simulink model "TSR_Scenario_005_cs"  (R2014b)
settings: Solver=ode5  SolverMode=SingleTasking  StartTime=0.0  StopTime=inf  FixedStep=1/100  RelTol=1e-3
PreLoadFcn:
  | mbxruntime.callbacks.PreLoadFcn(bdroot);
  | check_NUTS_defined;
  | 
  | assignin('base',['model_closed_' bdroot],false);
  | 
  | addpath('../includes_TSR/includes_TSR');
  | 
  | switch version('-release')
  | case {'2010a', '2010b', '2011a'}
  | addpath('../includes_TSR/ML2010b');
  | otherwise
  | addpath('../includes_TSR/ML2011b');
  | end
PostLoadFcn:
  | mbxruntime.callbacks.PostLoadFcn(bdroot);
InitFcn:
  | mbxruntime.callbacks.InitFcn(bdroot);
StartFcn:
  | mbxruntime.callbacks.StartFcn(bdroot);
StopFcn:
  | mbxruntime.callbacks.StopFcn(bdroot);
model workspace: external: MAT-File .\TSR_Scenario_005_cs_hws.mat (data not in the file)
undefined symbols (not defined in the file or in its folder): InitImageOutputDir, mbxruntime, OrientationPitch, OrientationRoll, PositionX, PositionY, PositionZ, tabledata, warningInitialVelocity, x0
undefined symbols (not defined in the file): SteeringColumn, SteeringWheel, TSR_Scenario_005_cs_00431f954bf6ed0a, TSR_Scenario_005_cs_02a6645fe307ce96, TSR_Scenario_005_cs_0e0d17e780cba748, TSR_Scenario_005_cs_0f94700004e304be, TSR_Scenario_005_cs_13e63084604f23c5, TSR_Scenario_005_cs_18da76569b226b1d, TSR_Scenario_005_cs_19a09eb0dceaf389, TSR_Scenario_005_cs_1d6b1ecf339da803, TSR_Scenario_005_cs_219485daa5a5d171, TSR_Scenario_005_cs_221c03cfb0670d1a, TSR_Scenario_005_cs_22611db63f83df91, TSR_Scenario_005_cs_24324341e1f0fdeb, TSR_Scenario_005_cs_248b5be6aaeb4a32, TSR_Scenario_005_cs_26d69342f02903e6, TSR_Scenario_005_cs_28d4639b4eb6a924, TSR_Scenario_005_cs_2a50646ef6121283, TSR_Scenario_005_cs_2addef8764f78195, TSR_Scenario_005_cs_2c78bb6e92f1c73d, TSR_Scenario_005_cs_330b013c7926b8c0, TSR_Scenario_005_cs_33ac55a3a4bfafc5, TSR_Scenario_005_cs_33d6442482a921b6, TSR_Scenario_005_cs_36fcc85960c1dc31, TSR_Scenario_005_cs_38acb22310967a91, TSR_Scenario_005_cs_3e8855054a9c05f5, TSR_Scenario_005_cs_43d01b44652f0f38, TSR_Scenario_005_cs_43d19ecb630bd754, TSR_Scenario_005_cs_4487c76a87b8c5f1, TSR_Scenario_005_cs_44ceee846c318dfb, TSR_Scenario_005_cs_450a3683cbfdd730, TSR_Scenario_005_cs_464618e49e37493a, TSR_Scenario_005_cs_4880b38df4698ab1, TSR_Scenario_005_cs_4a2b3c7d0abca22e, TSR_Scenario_005_cs_4bd204b8239d5406, TSR_Scenario_005_cs_4de8d67ffbf74a19, TSR_Scenario_005_cs_4f6170ee339e194e, TSR_Scenario_005_cs_50430c8166448bfc, TSR_Scenario_005_cs_53c8f6734eaacbd2, TSR_Scenario_005_cs_543db9a2ff458ebe, TSR_Scenario_005_cs_57976f30ab2edad5, TSR_Scenario_005_cs_5922fccf31372278, TSR_Scenario_005_cs_5a258c940bbe826b, TSR_Scenario_005_cs_6087cc283675db35, TSR_Scenario_005_cs_6246b869963d4acb, TSR_Scenario_005_cs_6352b9f9b72630f9, TSR_Scenario_005_cs_6559b64eceddc3ca, TSR_Scenario_005_cs_6832a8ea8fa66aa4, TSR_Scenario_005_cs_696d53dba69844e5, TSR_Scenario_005_cs_6cabbb37c4ac2dd1, TSR_Scenario_005_cs_6d528aa494c8a952, TSR_Scenario_005_cs_6d945b49f7234fd2, TSR_Scenario_005_cs_6e2ebc771acb2455, TSR_Scenario_005_cs_7897f864ad990cf0, TSR_Scenario_005_cs_7978c65fd141f076, TSR_Scenario_005_cs_7a9ba94120bbe2c7, TSR_Scenario_005_cs_7b108592703c2dc5, TSR_Scenario_005_cs_7cd2f5b09394b811, TSR_Scenario_005_cs_7e1904d085d8f37f, TSR_Scenario_005_cs_7e555208507e0618 ... (+95)
libraries: simulink_extras x59, PreScanSimulinkLibrary x43, simulink x29
(part 19 of 24)

== system TSR_Scenario_005_cs/Audi_A8_1/WheelDisplacement_Mux/WheelR0_Mux ==
  X [m] : Inport
  Y [m] : Inport  Port=2
  Z [m] : Inport  Port=3
  Roll [rad] : Inport  Port=4
  Pitch [rad] : Inport  Port=5
  Yaw [rad] : Inport  Port=6
  Bus Creator : BusCreator  Inputs=3  OutDataTypeStr=Bus: PRESCAN_XYZ_DATA
  Bus Creator1 : BusCreator  Inputs=3  OutDataTypeStr=Bus: PRESCAN_RPY_DATA
  Bus Creator2 : BusCreator  Inputs=2  OutDataTypeStr=Bus: PRESCAN_POSE_DATA
  Joint : Outport
  wires:
  Yaw [rad]/1 -> Bus Creator1/3  "Yaw"
  Bus Creator1/1 -> Bus Creator2/2  "ORIENTATION"
  Bus Creator/1 -> Bus Creator2/1  "POSITION"
  X [m]/1 -> Bus Creator/1  "X"
  Y [m]/1 -> Bus Creator/2  "Y"
  Z [m]/1 -> Bus Creator/3  "Z"
  Bus Creator2/1 -> Joint/1
  Roll [rad]/1 -> Bus Creator1/1  "Roll"
  Pitch [rad]/1 -> Bus Creator1/2  "Pitch"

== system TSR_Scenario_005_cs/Audi_A8_1/WheelDisplacement_Mux/WheelR1_Mux ==
  X [m] : Inport
  Y [m] : Inport  Port=2
  Z [m] : Inport  Port=3
  Roll [rad] : Inport  Port=4
  Pitch [rad] : Inport  Port=5
  Yaw [rad] : Inport  Port=6
  Bus Creator : BusCreator  Inputs=3  OutDataTypeStr=Bus: PRESCAN_XYZ_DATA
  Bus Creator1 : BusCreator  Inputs=3  OutDataTypeStr=Bus: PRESCAN_RPY_DATA
  Bus Creator2 : BusCreator  Inputs=2  OutDataTypeStr=Bus: PRESCAN_POSE_DATA
  Joint : Outport
  wires:
  Yaw [rad]/1 -> Bus Creator1/3  "Yaw"
  Bus Creator1/1 -> Bus Creator2/2  "ORIENTATION"
  Bus Creator/1 -> Bus Creator2/1  "POSITION"
  X [m]/1 -> Bus Creator/1  "X"
  Y [m]/1 -> Bus Creator/2  "Y"
  Z [m]/1 -> Bus Creator/3  "Z"
  Bus Creator2/1 -> Joint/1
  Roll [rad]/1 -> Bus Creator1/1  "Roll"
  Pitch [rad]/1 -> Bus Creator1/2  "Pitch"

== system TSR_Scenario_005_cs/BMW_X5_1/Dynamics_Empty/MuxState ==
  note: mode: Dynamics
  note: mode: Positioning
  note: mode: Dynamics
      | VelVEHICLE
      | wrt VEH
  note: AnglesVEHICLE
      | wrtGLOB
  note: For state mode 'Dynamic' positions
      | are not taken into account, as they
      | are computed by integrating velocity.
      | Click annotation for Help.
  x [m] : Inport  SampleTime=TimeStep
  y [m] : Inport  Port=2  SampleTime=TimeStep
  z [m] : Inport  Port=3  SampleTime=TimeStep
  dx [m/s] : Inport  Port=4  SampleTime=TimeStep
  dy [m/s] : Inport  Port=5  SampleTime=TimeStep
  dz [m/s] : Inport  Port=6  SampleTime=TimeStep
  R [rad] : Inport  Port=7  SampleTime=TimeStep
  P [rad] : Inport  Port=8  SampleTime=TimeStep
  Y [rad] : Inport  Port=9  SampleTime=TimeStep
  Constant : Constant  DisableCoverage=on  Value=positioningmode
  Discrete-Time Integrator : DiscreteIntegrator  SampleTime=TimeStep
  Ground : Ground
  Ground1 : Ground
  Mux1 : Mux  Inputs=[3 3]
  Mux2 : Mux  Inputs=3
  Mux3 : Mux  Inputs=3
  Mux4 : Mux  Inputs=3
  Mux5 : Mux  Inputs=[3 3]
  Mux6 : Mux  Inputs=[6 3]
  Switch : Switch  Threshold=0.5
  Transformation_BODY2GLOBAL : PreScanSimulinkLibrary/Simple_Vehicle_Dynamics/Chassis/MuxDynState/Transformation_BODY2GLOBAL
  mux3 : Mux  Inputs=3
  state : Outport
  wires:
  Constant/1 -> Switch/2
  Mux6/1 -> state/1
  Mux4/1 -> Mux1/1
  Mux5/1 -> Switch/3
  Mux1/1 -> Switch/1
  Switch/1 -> Mux6/1  "PosVeh wrt  GLOB"
  P [rad]/1 -> Mux3/2
  R [rad]/1 -> Mux3/1
  dz [m/s]/1 -> Mux2/3
  dy [m/s]/1 -> Mux2/2
  dx [m/s]/1 -> Mux2/1
  z [m]/1 -> Mux4/3
  y [m]/1 -> Mux4/2
  x [m]/1 -> Mux4/1
  Ground1/1 -> mux3/2  "pitch"
  Y [rad]/1 -> mux3/3, Mux3/3  "yaw"
  Mux3/1 -> Mux6/2
  Transformation_BODY2GLOBAL/1 -> Discrete-Time Integrator/1, Mux5/2  "VelVEH wrt  GLOB"
  mux3/1 -> Transformation_BODY2GLOBAL/2
  Ground/1 -> mux3/1  "roll"
  Mux2/1 -> Mux1/2, Transformation_BODY2GLOBAL/1
  Discrete-Time Integrator/1 -> Mux5/1  "PosVEH wrt  GLOB"

== system TSR_Scenario_005_cs/BMW_X5_1/Dynamics_Empty/STATE_BMW_X5_1 ==
  State : Inport  SampleTime=TimeStep
  Bus Creator : BusCreator  Inputs=15  OutDataTypeStr=Bus: PRESCAN_STATEACTUATORDATA  NonVirtualBus=on
  Constant : Constant  Value=0
  Demux : Demux  Outputs=15
  Mux : Mux  Inputs=3
  Mux1 : Mux  Inputs=3
  Mux2 : Mux  Inputs=3
  iniBODYAngles wrtVEH [rad] : Constant  Value=Roll0  SampleTime=TimeStep
  iniBODYAngles wrtVEH [rad]1 : Constant  Value=Pitch0  SampleTime=TimeStep
  iniVEHAngles wrtGLOB [rad] : Constant  Value=Yaw0  SampleTime=TimeStep
  iniVEHposition wrtGLOB [m] : Constant  Value=x0  SampleTime=TimeStep
  iniVEHposition wrtGLOB [m]1 : Constant  Value=y0  SampleTime=TimeStep
  iniVEHposition wrtGLOB [m]2 : Constant  Value=z0  SampleTime=TimeStep
  state2FullState : PreScanSimulinkLibrary/state2FullState  SystemSampleTime=-1
  StateBus : Outport  OutDataTypeStr=Bus: PRESCAN_STATEACTUATORDATA
  wires:
  Mux2/1 -> state2FullState/4
  iniVEHAngles wrtGLOB [rad]/1 -> Mux2/3
  Mux1/1 -> state2FullState/3
  Constant/1 -> Mux2/1, Mux2/2, Mux1/3
  iniBODYAngles wrtVEH [rad]1/1 -> Mux1/2
  iniBODYAngles wrtVEH [rad]/1 -> Mux1/1
  Mux/1 -> state2FullState/2
  iniVEHposition wrtGLOB [m]2/1 -> Mux/3
  iniVEHposition wrtGLOB [m]/1 -> Mux/1
  iniVEHposition wrtGLOB [m]1/1 -> Mux/2
  Demux/15 -> Bus Creator/15  "AngularVelocityYaw"
  Demux/14 -> Bus Creator/14  "AngularVelocityPitch"
  Demux/13 -> Bus Creator/13  "AngularVelocityRoll"
  Demux/12 -> Bus Creator/12  "OrientationYaw"
  Demux/11 -> Bus Creator/11  "OrientationPitch"
  Demux/10 -> Bus Creator/10  "OrientationRoll"
  Demux/9 -> Bus Creator/9  "AccelerationZ"
  Demux/8 -> Bus Creator/8  "AccelerationY"
  Demux/7 -> Bus Creator/7  "AccelerationX"
  Demux/6 -> Bus Creator/6  "VelocityZ"
  Demux/5 -> Bus Creator/5  "VelocityY"
  Demux/4 -> Bus Creator/4  "VelocityX"
  Demux/3 -> Bus Creator/3  "PositionZ"
  Demux/2 -> Bus Creator/2  "PositionY"
  Demux/1 -> Bus Creator/1  "PositionX"
  state2FullState/1 -> Demux/1
  State/1 -> state2FullState/1
  Bus Creator/1 -> StateBus/1

== system TSR_Scenario_005_cs/BMW_X5_1/SELF_Demux/compas converter ==
  rotz [rad] : Inport
  cart2compas : Subsystem
  rad2deg : Gain  Gain=180/pi
  heading [deg] : Outport
  wires:
  rad2deg/1 -> cart2compas/1(Angle [deg])
  rotz [rad]/1 -> rad2deg/1
  cart2compas/1(heading [deg]) -> heading [deg]/1

== system TSR_Scenario_005_cs/BMW_X5_2/Dynamics_Empty/MuxState ==
  note: mode: Dynamics
  note: mode: Positioning
  note: mode: Dynamics
      | VelVEHICLE
      | wrt VEH
  note: AnglesVEHICLE
      | wrtGLOB
  note: For state mode 'Dynamic' positions
      | are not taken into account, as they
      | are computed by integrating velocity.
      | Click annotation for Help.
  x [m] : Inport  SampleTime=TimeStep
  y [m] : Inport  Port=2  SampleTime=TimeStep
  z [m] : Inport  Port=3  SampleTime=TimeStep
  dx [m/s] : Inport  Port=4  SampleTime=TimeStep
  dy [m/s] : Inport  Port=5  SampleTime=TimeStep
  dz [m/s] : Inport  Port=6  SampleTime=TimeStep
  R [rad] : Inport  Port=7  SampleTime=TimeStep
  P [rad] : Inport  Port=8  SampleTime=TimeStep
  Y [rad] : Inport  Port=9  SampleTime=TimeStep
  Constant : Constant  DisableCoverage=on  Value=positioningmode
  Discrete-Time Integrator : DiscreteIntegrator  SampleTime=TimeStep
  Ground : Ground
  Ground1 : Ground
  Mux1 : Mux  Inputs=[3 3]
  Mux2 : Mux  Inputs=3
  Mux3 : Mux  Inputs=3
  Mux4 : Mux  Inputs=3
  Mux5 : Mux  Inputs=[3 3]
  Mux6 : Mux  Inputs=[6 3]
  Switch : Switch  Threshold=0.5
  Transformation_BODY2GLOBAL : PreScanSimulinkLibrary/Simple_Vehicle_Dynamics/Chassis/MuxDynState/Transformation_BODY2GLOBAL
  mux3 : Mux  Inputs=3
  state : Outport
  wires:
  Constant/1 -> Switch/2
  Mux6/1 -> state/1
  Mux4/1 -> Mux1/1
  Mux5/1 -> Switch/3
  Mux1/1 -> Switch/1
  Switch/1 -> Mux6/1  "PosVeh wrt  GLOB"
  P [rad]/1 -> Mux3/2
  R [rad]/1 -> Mux3/1
  dz [m/s]/1 -> Mux2/3
  dy [m/s]/1 -> Mux2/2
  dx [m/s]/1 -> Mux2/1
  z [m]/1 -> Mux4/3
  y [m]/1 -> Mux4/2
  x [m]/1 -> Mux4/1
  Ground1/1 -> mux3/2  "pitch"
  Y [rad]/1 -> mux3/3, Mux3/3  "yaw"
  Mux3/1 -> Mux6/2
  Transformation_BODY2GLOBAL/1 -> Discrete-Time Integrator/1, Mux5/2  "VelVEH wrt  GLOB"
  mux3/1 -> Transformation_BODY2GLOBAL/2
  Ground/1 -> mux3/1  "roll"
  Mux2/1 -> Mux1/2, Transformation_BODY2GLOBAL/1
  Discrete-Time Integrator/1 -> Mux5/1  "PosVEH wrt  GLOB"

== system TSR_Scenario_005_cs/BMW_X5_2/Dynamics_Empty/STATE_BMW_X5_2 ==
  State : Inport  SampleTime=TimeStep
  Bus Creator : BusCreator  Inputs=15  OutDataTypeStr=Bus: PRESCAN_STATEACTUATORDATA  NonVirtualBus=on
  Constant : Constant  Value=0
  Demux : Demux  Outputs=15
  Mux : Mux  Inputs=3
  Mux1 : Mux  Inputs=3
  Mux2 : Mux  Inputs=3
  iniBODYAngles wrtVEH [rad] : Constant  Value=Roll0  SampleTime=TimeStep
  iniBODYAngles wrtVEH [rad]1 : Constant  Value=Pitch0  SampleTime=TimeStep
  iniVEHAngles wrtGLOB [rad] : Constant  Value=Yaw0  SampleTime=TimeStep
  iniVEHposition wrtGLOB [m] : Constant  Value=x0  SampleTime=TimeStep
  iniVEHposition wrtGLOB [m]1 : Constant  Value=y0  SampleTime=TimeStep
  iniVEHposition wrtGLOB [m]2 : Constant  Value=z0  SampleTime=TimeStep
  state2FullState : PreScanSimulinkLibrary/state2FullState  SystemSampleTime=-1
  StateBus : Outport  OutDataTypeStr=Bus: PRESCAN_STATEACTUATORDATA
  wires:
  Mux2/1 -> state2FullState/4
  iniVEHAngles wrtGLOB [rad]/1 -> Mux2/3
  Mux1/1 -> state2FullState/3
  Constant/1 -> Mux2/1, Mux2/2, Mux1/3
  iniBODYAngles wrtVEH [rad]1/1 -> Mux1/2
  iniBODYAngles wrtVEH [rad]/1 -> Mux1/1
  Mux/1 -> state2FullState/2
  iniVEHposition wrtGLOB [m]2/1 -> Mux/3
  iniVEHposition wrtGLOB [m]/1 -> Mux/1
  iniVEHposition wrtGLOB [m]1/1 -> Mux/2
  Demux/15 -> Bus Creator/15  "AngularVelocityYaw"
  Demux/14 -> Bus Creator/14  "AngularVelocityPitch"
  Demux/13 -> Bus Creator/13  "AngularVelocityRoll"
  Demux/12 -> Bus Creator/12  "OrientationYaw"
  Demux/11 -> Bus Creator/11  "OrientationPitch"
  Demux/10 -> Bus Creator/10  "OrientationRoll"
  Demux/9 -> Bus Creator/9  "AccelerationZ"
  Demux/8 -> Bus Creator/8  "AccelerationY"
  Demux/7 -> Bus Creator/7  "AccelerationX"
  Demux/6 -> Bus Creator/6  "VelocityZ"
  Demux/5 -> Bus Creator/5  "VelocityY"
  Demux/4 -> Bus Creator/4  "VelocityX"
  Demux/3 -> Bus Creator/3  "PositionZ"
  Demux/2 -> Bus Creator/2  "PositionY"
  Demux/1 -> Bus Creator/1  "PositionX"
  state2FullState/1 -> Demux/1
  State/1 -> state2FullState/1
  Bus Creator/1 -> StateBus/1

== system TSR_Scenario_005_cs/BMW_X5_2/SELF_Demux/compas converter ==
  rotz [rad] : Inport
  cart2compas : Subsystem
  rad2deg : Gain  Gain=180/pi
  heading [deg] : Outport
  wires:
  rad2deg/1 -> cart2compas/1(Angle [deg])
  rotz [rad]/1 -> rad2deg/1
  cart2compas/1(heading [deg]) -> heading [deg]/1

== system TSR_Scenario_005_cs/BMW_X5_3/Dynamics_Empty/MuxState ==
  note: mode: Dynamics
  note: mode: Positioning
  note: mode: Dynamics
      | VelVEHICLE
      | wrt VEH
  note: AnglesVEHICLE
      | wrtGLOB
  note: For state mode 'Dynamic' positions
      | are not taken into account, as they
      | are computed by integrating velocity.
      | Click annotation for Help.
  x [m] : Inport  SampleTime=TimeStep
  y [m] : Inport  Port=2  SampleTime=TimeStep
  z [m] : Inport  Port=3  SampleTime=TimeStep
  dx [m/s] : Inport  Port=4  SampleTime=TimeStep
  dy [m/s] : Inport  Port=5  SampleTime=TimeStep
  dz [m/s] : Inport  Port=6  SampleTime=TimeStep
  R [rad] : Inport  Port=7  SampleTime=TimeStep
  P [rad] : Inport  Port=8  SampleTime=TimeStep
  Y [rad] : Inport  Port=9  SampleTime=TimeStep
  Constant : Constant  DisableCoverage=on  Value=positioningmode
  Discrete-Time Integrator : DiscreteIntegrator  SampleTime=TimeStep
  Ground : Ground
  Ground1 : Ground
  Mux1 : Mux  Inputs=[3 3]
  Mux2 : Mux  Inputs=3
  Mux3 : Mux  Inputs=3
  Mux4 : Mux  Inputs=3
  Mux5 : Mux  Inputs=[3 3]
  Mux6 : Mux  Inputs=[6 3]
  Switch : Switch  Threshold=0.5
  Transformation_BODY2GLOBAL : PreScanSimulinkLibrary/Simple_Vehicle_Dynamics/Chassis/MuxDynState/Transformation_BODY2GLOBAL
  mux3 : Mux  Inputs=3
  state : Outport
  wires:
  Constant/1 -> Switch/2
  Mux6/1 -> state/1
  Mux4/1 -> Mux1/1
  Mux5/1 -> Switch/3
  Mux1/1 -> Switch/1
  Switch/1 -> Mux6/1  "PosVeh wrt  GLOB"
  P [rad]/1 -> Mux3/2
  R [rad]/1 -> Mux3/1
  dz [m/s]/1 -> Mux2/3
  dy [m/s]/1 -> Mux2/2
  dx [m/s]/1 -> Mux2/1
  z [m]/1 -> Mux4/3
  y [m]/1 -> Mux4/2
  x [m]/1 -> Mux4/1
  Ground1/1 -> mux3/2  "pitch"
  Y [rad]/1 -> mux3/3, Mux3/3  "yaw"
  Mux3/1 -> Mux6/2
  Transformation_BODY2GLOBAL/1 -> Discrete-Time Integrator/1, Mux5/2  "VelVEH wrt  GLOB"
  mux3/1 -> Transformation_BODY2GLOBAL/2
  Ground/1 -> mux3/1  "roll"
  Mux2/1 -> Mux1/2, Transformation_BODY2GLOBAL/1
  Discrete-Time Integrator/1 -> Mux5/1  "PosVEH wrt  GLOB"

== system TSR_Scenario_005_cs/BMW_X5_3/Dynamics_Empty/STATE_BMW_X5_3 ==
  State : Inport  SampleTime=TimeStep
  Bus Creator : BusCreator  Inputs=15  OutDataTypeStr=Bus: PRESCAN_STATEACTUATORDATA  NonVirtualBus=on
  Constant : Constant  Value=0
  Demux : Demux  Outputs=15
  Mux : Mux  Inputs=3
  Mux1 : Mux  Inputs=3
  Mux2 : Mux  Inputs=3
  iniBODYAngles wrtVEH [rad] : Constant  Value=Roll0  SampleTime=TimeStep
  iniBODYAngles wrtVEH [rad]1 : Constant  Value=Pitch0  SampleTime=TimeStep
  iniVEHAngles wrtGLOB [rad] : Constant  Value=Yaw0  SampleTime=TimeStep
  iniVEHposition wrtGLOB [m] : Constant  Value=x0  SampleTime=TimeStep
  iniVEHposition wrtGLOB [m]1 : Constant  Value=y0  SampleTime=TimeStep
  iniVEHposition wrtGLOB [m]2 : Constant  Value=z0  SampleTime=TimeStep
  state2FullState : PreScanSimulinkLibrary/state2FullState  SystemSampleTime=-1
  StateBus : Outport  OutDataTypeStr=Bus: PRESCAN_STATEACTUATORDATA
  wires:
  Mux2/1 -> state2FullState/4
  iniVEHAngles wrtGLOB [rad]/1 -> Mux2/3
  Mux1/1 -> state2FullState/3
  Constant/1 -> Mux2/1, Mux2/2, Mux1/3
  iniBODYAngles wrtVEH [rad]1/1 -> Mux1/2
  iniBODYAngles wrtVEH [rad]/1 -> Mux1/1
  Mux/1 -> state2FullState/2
  iniVEHposition wrtGLOB [m]2/1 -> Mux/3
  iniVEHposition wrtGLOB [m]/1 -> Mux/1
  iniVEHposition wrtGLOB [m]1/1 -> Mux/2
  Demux/15 -> Bus Creator/15  "AngularVelocityYaw"
  Demux/14 -> Bus Creator/14  "AngularVelocityPitch"
  Demux/13 -> Bus Creator/13  "AngularVelocityRoll"
  Demux/12 -> Bus Creator/12  "OrientationYaw"
  Demux/11 -> Bus Creator/11  "OrientationPitch"
  Demux/10 -> Bus Creator/10  "OrientationRoll"
  Demux/9 -> Bus Creator/9  "AccelerationZ"
  Demux/8 -> Bus Creator/8  "AccelerationY"
  Demux/7 -> Bus Creator/7  "AccelerationX"
  Demux/6 -> Bus Creator/6  "VelocityZ"
  Demux/5 -> Bus Creator/5  "VelocityY"
  Demux/4 -> Bus Creator/4  "VelocityX"
  Demux/3 -> Bus Creator/3  "PositionZ"
  Demux/2 -> Bus Creator/2  "PositionY"
  Demux/1 -> Bus Creator/1  "PositionX"
  state2FullState/1 -> Demux/1
  State/1 -> state2FullState/1
  Bus Creator/1 -> StateBus/1

== system TSR_Scenario_005_cs/BMW_X5_3/SELF_Demux/compas converter ==
  rotz [rad] : Inport
  cart2compas : Subsystem
  rad2deg : Gain  Gain=180/pi
  heading [deg] : Outport
  wires:
  rad2deg/1 -> cart2compas/1(Angle [deg])
  rotz [rad]/1 -> rad2deg/1
  cart2compas/1(heading [deg]) -> heading [deg]/1

== system TSR_Scenario_005_cs/BMW_Z3_1/Dynamics_Empty/MuxState ==
  note: mode: Dynamics
  note: mode: Positioning
  note: mode: Dynamics
      | VelVEHICLE
      | wrt VEH
  note: AnglesVEHICLE
      | wrtGLOB
  note: For state mode 'Dynamic' positions
      | are not taken into account, as they
      | are computed by integrating velocity.
      | Click annotation for Help.
  x [m] : Inport  SampleTime=TimeStep
  y [m] : Inport  Port=2  SampleTime=TimeStep
  z [m] : Inport  Port=3  SampleTime=TimeStep
  dx [m/s] : Inport  Port=4  SampleTime=TimeStep
  dy [m/s] : Inport  Port=5  SampleTime=TimeStep
  dz [m/s] : Inport  Port=6  SampleTime=TimeStep
  R [rad] : Inport  Port=7  SampleTime=TimeStep
  P [rad] : Inport  Port=8  SampleTime=TimeStep
  Y [rad] : Inport  Port=9  SampleTime=TimeStep
  Constant : Constant  DisableCoverage=on  Value=positioningmode
  Discrete-Time Integrator : DiscreteIntegrator  SampleTime=TimeStep
  Ground : Ground
  Ground1 : Ground
  Mux1 : Mux  Inputs=[3 3]
  Mux2 : Mux  Inputs=3
  Mux3 : Mux  Inputs=3
  Mux4 : Mux  Inputs=3
  Mux5 : Mux  Inputs=[3 3]
  Mux6 : Mux  Inputs=[6 3]
  Switch : Switch  Threshold=0.5
  Transformation_BODY2GLOBAL : PreScanSimulinkLibrary/Simple_Vehicle_Dynamics/Chassis/MuxDynState/Transformation_BODY2GLOBAL
  mux3 : Mux  Inputs=3
  state : Outport
  wires:
  Constant/1 -> Switch/2
  Mux6/1 -> state/1
  Mux4/1 -> Mux1/1
  Mux5/1 -> Switch/3
  Mux1/1 -> Switch/1
  Switch/1 -> Mux6/1  "PosVeh wrt  GLOB"
  P [rad]/1 -> Mux3/2
  R [rad]/1 -> Mux3/1
  dz [m/s]/1 -> Mux2/3
  dy [m/s]/1 -> Mux2/2
  dx [m/s]/1 -> Mux2/1
  z [m]/1 -> Mux4/3
  y [m]/1 -> Mux4/2
  x [m]/1 -> Mux4/1
  Ground1/1 -> mux3/2  "pitch"
  Y [rad]/1 -> mux3/3, Mux3/3  "yaw"
  Mux3/1 -> Mux6/2
  Transformation_BODY2GLOBAL/1 -> Discrete-Time Integrator/1, Mux5/2  "VelVEH wrt  GLOB"
  mux3/1 -> Transformation_BODY2GLOBAL/2
  Ground/1 -> mux3/1  "roll"
  Mux2/1 -> Mux1/2, Transformation_BODY2GLOBAL/1
  Discrete-Time Integrator/1 -> Mux5/1  "PosVEH wrt  GLOB"

== system TSR_Scenario_005_cs/BMW_Z3_1/Dynamics_Empty/STATE_BMW_Z3_1 ==
  State : Inport  SampleTime=TimeStep
  Bus Creator : BusCreator  Inputs=15  OutDataTypeStr=Bus: PRESCAN_STATEACTUATORDATA  NonVirtualBus=on
  Constant : Constant  Value=0
  Demux : Demux  Outputs=15
  Mux : Mux  Inputs=3
  Mux1 : Mux  Inputs=3
  Mux2 : Mux  Inputs=3
  iniBODYAngles wrtVEH [rad] : Constant  Value=Roll0  SampleTime=TimeStep
  iniBODYAngles wrtVEH [rad]1 : Constant  Value=Pitch0  SampleTime=TimeStep
  iniVEHAngles wrtGLOB [rad] : Constant  Value=Yaw0  SampleTime=TimeStep
  iniVEHposition wrtGLOB [m] : Constant  Value=x0  SampleTime=TimeStep
  iniVEHposition wrtGLOB [m]1 : Constant  Value=y0  SampleTime=TimeStep
  iniVEHposition wrtGLOB [m]2 : Constant  Value=z0  SampleTime=TimeStep
  state2FullState : PreScanSimulinkLibrary/state2FullState  SystemSampleTime=-1
  StateBus : Outport  OutDataTypeStr=Bus: PRESCAN_STATEACTUATORDATA
  wires:
  Mux2/1 -> state2FullState/4
  iniVEHAngles wrtGLOB [rad]/1 -> Mux2/3
  Mux1/1 -> state2FullState/3
  Constant/1 -> Mux2/1, Mux2/2, Mux1/3
  iniBODYAngles wrtVEH [rad]1/1 -> Mux1/2
  iniBODYAngles wrtVEH [rad]/1 -> Mux1/1
  Mux/1 -> state2FullState/2
  iniVEHposition wrtGLOB [m]2/1 -> Mux/3
  iniVEHposition wrtGLOB [m]/1 -> Mux/1
  iniVEHposition wrtGLOB [m]1/1 -> Mux/2
  Demux/15 -> Bus Creator/15  "AngularVelocityYaw"
  Demux/14 -> Bus Creator/14  "AngularVelocityPitch"
  Demux/13 -> Bus Creator/13  "AngularVelocityRoll"
  Demux/12 -> Bus Creator/12  "OrientationYaw"
  Demux/11 -> Bus Creator/11  "OrientationPitch"
  Demux/10 -> Bus Creator/10  "OrientationRoll"
  Demux/9 -> Bus Creator/9  "AccelerationZ"
  Demux/8 -> Bus Creator/8  "AccelerationY"
  Demux/7 -> Bus Creator/7  "AccelerationX"
  Demux/6 -> Bus Creator/6  "VelocityZ"
  Demux/5 -> Bus Creator/5  "VelocityY"
  Demux/4 -> Bus Creator/4  "VelocityX"
  Demux/3 -> Bus Creator/3  "PositionZ"
  Demux/2 -> Bus Creator/2  "PositionY"
  Demux/1 -> Bus Creator/1  "PositionX"
  state2FullState/1 -> Demux/1
  State/1 -> state2FullState/1
  Bus Creator/1 -> StateBus/1

== system TSR_Scenario_005_cs/BMW_Z3_1/SELF_Demux/compas converter ==
  rotz [rad] : Inport
  cart2compas : Subsystem
  rad2deg : Gain  Gain=180/pi
  heading [deg] : Outport
  wires:
  rad2deg/1 -> cart2compas/1(Angle [deg])
  rotz [rad]/1 -> rad2deg/1
  cart2compas/1(heading [deg]) -> heading [deg]/1

== system TSR_Scenario_005_cs/CarTrailer_SingleAxle_1/SELF_Demux/compas converter ==
  rotz [rad] : Inport
  cart2compas : Subsystem
  rad2deg : Gain  Gain=180/pi
  heading [deg] : Outport
  wires:
  rad2deg/1 -> cart2compas/1(Angle [deg])
  rotz [rad]/1 -> rad2deg/1
  cart2compas/1(heading [deg]) -> heading [deg]/1

== system TSR_Scenario_005_cs/Citroen_C3_1/Dynamics_Empty/MuxState ==
  note: mode: Dynamics
  note: mode: Positioning
  note: mode: Dynamics
      | VelVEHICLE
      | wrt VEH
  note: AnglesVEHICLE
      | wrtGLOB
  note: For state mode 'Dynamic' positions
      | are not taken into account, as they
      | are computed by integrating velocity.
      | Click annotation for Help.
  x [m] : Inport  SampleTime=TimeStep
  y [m] : Inport  Port=2  SampleTime=TimeStep
  z [m] : Inport  Port=3  SampleTime=TimeStep
  dx [m/s] : Inport  Port=4  SampleTime=TimeStep
  dy [m/s] : Inport  Port=5  SampleTime=TimeStep
  dz [m/s] : Inport  Port=6  SampleTime=TimeStep
  R [rad] : Inport  Port=7  SampleTime=TimeStep
  P [rad] : Inport  Port=8  SampleTime=TimeStep
  Y [rad] : Inport  Port=9  SampleTime=TimeStep
  Constant : Constant  DisableCoverage=on  Value=positioningmode
  Discrete-Time Integrator : DiscreteIntegrator  SampleTime=TimeStep
  Ground : Ground
  Ground1 : Ground
  Mux1 : Mux  Inputs=[3 3]
  Mux2 : Mux  Inputs=3
  Mux3 : Mux  Inputs=3
  Mux4 : Mux  Inputs=3
  Mux5 : Mux  Inputs=[3 3]
  Mux6 : Mux  Inputs=[6 3]
  Switch : Switch  Threshold=0.5
  Transformation_BODY2GLOBAL : PreScanSimulinkLibrary/Simple_Vehicle_Dynamics/Chassis/MuxDynState/Transformation_BODY2GLOBAL
  mux3 : Mux  Inputs=3
  state : Outport
  wires:
  Constant/1 -> Switch/2
  Mux6/1 -> state/1
  Mux4/1 -> Mux1/1
  Mux5/1 -> Switch/3
  Mux1/1 -> Switch/1
  Switch/1 -> Mux6/1  "PosVeh wrt  GLOB"
  P [rad]/1 -> Mux3/2
  R [rad]/1 -> Mux3/1
  dz [m/s]/1 -> Mux2/3
  dy [m/s]/1 -> Mux2/2
  dx [m/s]/1 -> Mux2/1
  z [m]/1 -> Mux4/3
  y [m]/1 -> Mux4/2
  x [m]/1 -> Mux4/1
  Ground1/1 -> mux3/2  "pitch"
  Y [rad]/1 -> mux3/3, Mux3/3  "yaw"
  Mux3/1 -> Mux6/2
  Transformation_BODY2GLOBAL/1 -> Discrete-Time Integrator/1, Mux5/2  "VelVEH wrt  GLOB"
  mux3/1 -> Transformation_BODY2GLOBAL/2
  Ground/1 -> mux3/1  "roll"
  Mux2/1 -> Mux1/2, Transformation_BODY2GLOBAL/1
  Discrete-Time Integrator/1 -> Mux5/1  "PosVEH wrt  GLOB"

== system TSR_Scenario_005_cs/Citroen_C3_1/Dynamics_Empty/STATE_Citroen_C3_1 ==
  State : Inport  SampleTime=TimeStep
  Bus Creator : BusCreator  Inputs=15  OutDataTypeStr=Bus: PRESCAN_STATEACTUATORDATA  NonVirtualBus=on
  Constant : Constant  Value=0
  Demux : Demux  Outputs=15
  Mux : Mux  Inputs=3
  Mux1 : Mux  Inputs=3
  Mux2 : Mux  Inputs=3
  iniBODYAngles wrtVEH [rad] : Constant  Value=Roll0  SampleTime=TimeStep
  iniBODYAngles wrtVEH [rad]1 : Constant  Value=Pitch0  SampleTime=TimeStep
  iniVEHAngles wrtGLOB [rad] : Constant  Value=Yaw0  SampleTime=TimeStep
  iniVEHposition wrtGLOB [m] : Constant  Value=x0  SampleTime=TimeStep
  iniVEHposition wrtGLOB [m]1 : Constant  Value=y0  SampleTime=TimeStep
  iniVEHposition wrtGLOB [m]2 : Constant  Value=z0  SampleTime=TimeStep
  state2FullState : PreScanSimulinkLibrary/state2FullState  SystemSampleTime=-1
  StateBus : Outport  OutDataTypeStr=Bus: PRESCAN_STATEACTUATORDATA
  wires:
  Mux2/1 -> state2FullState/4
  iniVEHAngles wrtGLOB [rad]/1 -> Mux2/3
  Mux1/1 -> state2FullState/3
  Constant/1 -> Mux2/1, Mux2/2, Mux1/3
  iniBODYAngles wrtVEH [rad]1/1 -> Mux1/2
  iniBODYAngles wrtVEH [rad]/1 -> Mux1/1
  Mux/1 -> state2FullState/2
  iniVEHposition wrtGLOB [m]2/1 -> Mux/3
  iniVEHposition wrtGLOB [m]/1 -> Mux/1
  iniVEHposition wrtGLOB [m]1/1 -> Mux/2
  Demux/15 -> Bus Creator/15  "AngularVelocityYaw"
  Demux/14 -> Bus Creator/14  "AngularVelocityPitch"
  Demux/13 -> Bus Creator/13  "AngularVelocityRoll"
  Demux/12 -> Bus Creator/12  "OrientationYaw"
  Demux/11 -> Bus Creator/11  "OrientationPitch"
  Demux/10 -> Bus Creator/10  "OrientationRoll"
  Demux/9 -> Bus Creator/9  "AccelerationZ"
  Demux/8 -> Bus Creator/8  "AccelerationY"
  Demux/7 -> Bus Creator/7  "AccelerationX"
  Demux/6 -> Bus Creator/6  "VelocityZ"
  Demux/5 -> Bus Creator/5  "VelocityY"
  Demux/4 -> Bus Creator/4  "VelocityX"
  Demux/3 -> Bus Creator/3  "PositionZ"
  Demux/2 -> Bus Creator/2  "PositionY"
  Demux/1 -> Bus Creator/1  "PositionX"
  state2FullState/1 -> Demux/1
  State/1 -> state2FullState/1
  Bus Creator/1 -> StateBus/1

== system TSR_Scenario_005_cs/Citroen_C3_1/SELF_Demux/compas converter ==
  rotz [rad] : Inport
  cart2compas : Subsystem
  rad2deg : Gain  Gain=180/pi
  heading [deg] : Outport
  wires:
  rad2deg/1 -> cart2compas/1(Angle [deg])
  rotz [rad]/1 -> rad2deg/1
  cart2compas/1(heading [deg]) -> heading [deg]/1

== system TSR_Scenario_005_cs/Daf_95_1/SELF_Demux/compas converter ==
  rotz [rad] : Inport
  cart2compas : Subsystem
  rad2deg : Gain  Gain=180/pi
  heading [deg] : Outport
  wires:
  rad2deg/1 -> cart2compas/1(Angle [deg])
  rotz [rad]/1 -> rad2deg/1
  cart2compas/1(heading [deg]) -> heading [deg]/1

== system TSR_Scenario_005_cs/Female_RegularAni_1/Animation/animation mode ==
  vel : Inport
  Data Type Conversion : DataTypeConversion  OutDataTypeStr=double
  Fcn : Fcn  Expr=sqrt(u(1)^2+u(2)^2+u(3)^2)
  Running : simulink/Logic and Bit Operations/Compare To Constant  relop=>=  const=MWS  OutDataTypeStr=uint8  ZeroCross=off
  Sum : Sum  Inputs=|++
  Walking : simulink/Logic and Bit Operations/Compare To Zero  relop=~=  OutDataTypeStr=uint8  ZeroCross=off
  mode : Outport
  wires:
  vel/1 -> Fcn/1
  Sum/1 -> Data Type Conversion/1
  Walking/1 -> Sum/1
  Running/1 -> Sum/2
  Fcn/1 -> Walking/1, Running/1
  Data Type Conversion/1 -> mode/1

== system TSR_Scenario_005_cs/Female_RegularAni_1/Animation/elapsed track ==
  vel : Inport
  Discrete-Time Integrator : DiscreteIntegrator  SampleTime=-1
  Fcn : Fcn  Expr=sqrt(u(1)^2 + u(2)^2 + u(3)^2)
  s : Outport
  wires:
  Fcn/1 -> Discrete-Time Integrator/1
  vel/1 -> Fcn/1
  Discrete-Time Integrator/1 -> s/1

== system TSR_Scenario_005_cs/Female_RegularAni_1/SELF_Demux/compas converter ==
  rotz [rad] : Inport
  cart2compas : Subsystem
  rad2deg : Gain  Gain=180/pi
  heading [deg] : Outport
  wires:
  rad2deg/1 -> cart2compas/1(Angle [deg])
  rotz [rad]/1 -> rad2deg/1
  cart2compas/1(heading [deg]) -> heading [deg]/1

== system TSR_Scenario_005_cs/Female_Regular_wBuggy_1/Animation/animation mode ==
  vel : Inport
  Data Type Conversion : DataTypeConversion  OutDataTypeStr=int32
  Fcn : Fcn  Expr=u(1)^2+u(2)^2+u(3)^2
  Walking : simulink/Logic and Bit Operations/Compare To Zero  relop=~=  OutDataTypeStr=uint8  ZeroCross=off
  mode : Outport
  wires:
  Data Type Conversion/1 -> mode/1
  Walking/1 -> Data Type Conversion/1
  Fcn/1 -> Walking/1
  vel/1 -> Fcn/1

== system TSR_Scenario_005_cs/Female_Regular_wBuggy_1/Animation/elapsed track ==
  vel : Inport
  Discrete-Time Integrator : DiscreteIntegrator  SampleTime=-1
  Fcn : Fcn  Expr=sqrt(u(1)^2 + u(2)^2 + u(3)^2)
  s : Outport
  wires:
  Discrete-Time Integrator/1 -> s/1
  vel/1 -> Fcn/1
  Fcn/1 -> Discrete-Time Integrator/1

== system TSR_Scenario_005_cs/Female_Regular_wBuggy_1/Dynamics_Empty/MuxState ==
  note: mode: Dynamics
  note: mode: Positioning
  note: mode: Dynamics
      | VelVEHICLE
      | wrt VEH
  note: AnglesVEHICLE
      | wrtGLOB
  note: For state mode 'Dynamic' positions
      | are not taken into account, as they
      | are computed by integrating velocity.
      | Click annotation for Help.
  x [m] : Inport  SampleTime=TimeStep
  y [m] : Inport  Port=2  SampleTime=TimeStep
  z [m] : Inport  Port=3  SampleTime=TimeStep
  dx [m/s] : Inport  Port=4  SampleTime=TimeStep
  dy [m/s] : Inport  Port=5  SampleTime=TimeStep
  dz [m/s] : Inport  Port=6  SampleTime=TimeStep
  R [rad] : Inport  Port=7  SampleTime=TimeStep
  P [rad] : Inport  Port=8  SampleTime=TimeStep
  Y [rad] : Inport  Port=9  SampleTime=TimeStep
  Constant : Constant  DisableCoverage=on  Value=positioningmode
  Discrete-Time Integrator : DiscreteIntegrator  SampleTime=TimeStep
  Ground : Ground
  Ground1 : Ground
  Mux1 : Mux  Inputs=[3 3]
  Mux2 : Mux  Inputs=3
  Mux3 : Mux  Inputs=3
  Mux4 : Mux  Inputs=3
  Mux5 : Mux  Inputs=[3 3]
  Mux6 : Mux  Inputs=[6 3]
  Switch : Switch  Threshold=0.5
  Transformation_BODY2GLOBAL : PreScanSimulinkLibrary/Simple_Vehicle_Dynamics/Chassis/MuxDynState/Transformation_BODY2GLOBAL
  mux3 : Mux  Inputs=3
  state : Outport
  wires:
  Constant/1 -> Switch/2
  Mux6/1 -> state/1
  Mux4/1 -> Mux1/1
  Mux5/1 -> Switch/3
  Mux1/1 -> Switch/1
  Switch/1 -> Mux6/1  "PosVeh wrt  GLOB"
  P [rad]/1 -> Mux3/2
  R [rad]/1 -> Mux3/1
  dz [m/s]/1 -> Mux2/3
  dy [m/s]/1 -> Mux2/2
  dx [m/s]/1 -> Mux2/1
  z [m]/1 -> Mux4/3
  y [m]/1 -> Mux4/2
  x [m]/1 -> Mux4/1
  Ground1/1 -> mux3/2  "pitch"
  Y [rad]/1 -> mux3/3, Mux3/3  "yaw"
  Mux3/1 -> Mux6/2
  Transformation_BODY2GLOBAL/1 -> Discrete-Time Integrator/1, Mux5/2  "VelVEH wrt  GLOB"
  mux3/1 -> Transformation_BODY2GLOBAL/2
  Ground/1 -> mux3/1  "roll"
  Mux2/1 -> Mux1/2, Transformation_BODY2GLOBAL/1
  Discrete-Time Integrator/1 -> Mux5/1  "PosVEH wrt  GLOB"

== system TSR_Scenario_005_cs/Female_Regular_wBuggy_1/Dynamics_Empty/STATE_Female_Regular_wBuggy_1 ==
  State : Inport  SampleTime=TimeStep
  Bus Creator : BusCreator  Inputs=15  OutDataTypeStr=Bus: PRESCAN_STATEACTUATORDATA  NonVirtualBus=on
  Constant : Constant  Value=0
  Demux : Demux  Outputs=15
  Mux : Mux  Inputs=3
  Mux1 : Mux  Inputs=3
  Mux2 : Mux  Inputs=3
  iniBODYAngles wrtVEH [rad] : Constant  Value=Roll0  SampleTime=TimeStep
  iniBODYAngles wrtVEH [rad]1 : Constant  Value=Pitch0  SampleTime=TimeStep
  iniVEHAngles wrtGLOB [rad] : Constant  Value=Yaw0  SampleTime=TimeStep
  iniVEHposition wrtGLOB [m] : Constant  Value=x0  SampleTime=TimeStep
  iniVEHposition wrtGLOB [m]1 : Constant  Value=y0  SampleTime=TimeStep
  iniVEHposition wrtGLOB [m]2 : Constant  Value=z0  SampleTime=TimeStep
  state2FullState : PreScanSimulinkLibrary/state2FullState  SystemSampleTime=-1
  StateBus : Outport  OutDataTypeStr=Bus: PRESCAN_STATEACTUATORDATA
  wires:
  Mux2/1 -> state2FullState/4
  iniVEHAngles wrtGLOB [rad]/1 -> Mux2/3
  Mux1/1 -> state2FullState/3
  Constant/1 -> Mux2/1, Mux2/2, Mux1/3
  iniBODYAngles wrtVEH [rad]1/1 -> Mux1/2
  iniBODYAngles wrtVEH [rad]/1 -> Mux1/1
  Mux/1 -> state2FullState/2
  iniVEHposition wrtGLOB [m]2/1 -> Mux/3
  iniVEHposition wrtGLOB [m]/1 -> Mux/1
  iniVEHposition wrtGLOB [m]1/1 -> Mux/2
  Demux/15 -> Bus Creator/15  "AngularVelocityYaw"
  Demux/14 -> Bus Creator/14  "AngularVelocityPitch"
  Demux/13 -> Bus Creator/13  "AngularVelocityRoll"
  Demux/12 -> Bus Creator/12  "OrientationYaw"
  Demux/11 -> Bus Creator/11  "OrientationPitch"
  Demux/10 -> Bus Creator/10  "OrientationRoll"
  Demux/9 -> Bus Creator/9  "AccelerationZ"
  Demux/8 -> Bus Creator/8  "AccelerationY"
  Demux/7 -> Bus Creator/7  "AccelerationX"
  Demux/6 -> Bus Creator/6  "VelocityZ"
  Demux/5 -> Bus Creator/5  "VelocityY"
  Demux/4 -> Bus Creator/4  "VelocityX"
  Demux/3 -> Bus Creator/3  "PositionZ"
  Demux/2 -> Bus Creator/2  "PositionY"
  Demux/1 -> Bus Creator/1  "PositionX"
  state2FullState/1 -> Demux/1
  State/1 -> state2FullState/1
  Bus Creator/1 -> StateBus/1

== system TSR_Scenario_005_cs/Female_Regular_wBuggy_1/SELF_Demux/compas converter ==
  rotz [rad] : Inport
  cart2compas : Subsystem
  rad2deg : Gain  Gain=180/pi
  heading [deg] : Outport
  wires:
  rad2deg/1 -> cart2compas/1(Angle [deg])
  rotz [rad]/1 -> rad2deg/1
  cart2compas/1(heading [deg]) -> heading [deg]/1

== system TSR_Scenario_005_cs/Fiat_Bravo_1/Dynamics_Empty/MuxState ==
  note: mode: Dynamics
  note: mode: Positioning
  note: mode: Dynamics
      | VelVEHICLE
      | wrt VEH
  note: AnglesVEHICLE
      | wrtGLOB
  note: For state mode 'Dynamic' positions
      | are not taken into account, as they
      | are computed by integrating velocity.
      | Click annotation for Help.
  x [m] : Inport  SampleTime=TimeStep
  y [m] : Inport  Port=2  SampleTime=TimeStep
  z [m] : Inport  Port=3  SampleTime=TimeStep
  dx [m/s] : Inport  Port=4  SampleTime=TimeStep
  dy [m/s] : Inport  Port=5  SampleTime=TimeStep
  dz [m/s] : Inport  Port=6  SampleTime=TimeStep
  R [rad] : Inport  Port=7  SampleTime=TimeStep
  P [rad] : Inport  Port=8  SampleTime=TimeStep
  Y [rad] : Inport  Port=9  SampleTime=TimeStep
  Constant : Constant  DisableCoverage=on  Value=positioningmode
  Discrete-Time Integrator : DiscreteIntegrator  SampleTime=TimeStep
  Ground : Ground
  Ground1 : Ground
  Mux1 : Mux  Inputs=[3 3]
  Mux2 : Mux  Inputs=3
  Mux3 : Mux  Inputs=3
  Mux4 : Mux  Inputs=3
  Mux5 : Mux  Inputs=[3 3]
  Mux6 : Mux  Inputs=[6 3]
  Switch : Switch  Threshold=0.5
  Transformation_BODY2GLOBAL : PreScanSimulinkLibrary/Simple_Vehicle_Dynamics/Chassis/MuxDynState/Transformation_BODY2GLOBAL
  mux3 : Mux  Inputs=3
  state : Outport
  wires:
  Constant/1 -> Switch/2
  Mux6/1 -> state/1
  Mux4/1 -> Mux1/1
  Mux5/1 -> Switch/3
  Mux1/1 -> Switch/1
  Switch/1 -> Mux6/1  "PosVeh wrt  GLOB"
  P [rad]/1 -> Mux3/2
  R [rad]/1 -> Mux3/1
  dz [m/s]/1 -> Mux2/3
  dy [m/s]/1 -> Mux2/2
  dx [m/s]/1 -> Mux2/1
  z [m]/1 -> Mux4/3
  y [m]/1 -> Mux4/2
  x [m]/1 -> Mux4/1
  Ground1/1 -> mux3/2  "pitch"
  Y [rad]/1 -> mux3/3, Mux3/3  "yaw"
  Mux3/1 -> Mux6/2
  Transformation_BODY2GLOBAL/1 -> Discrete-Time Integrator/1, Mux5/2  "VelVEH wrt  GLOB"
  mux3/1 -> Transformation_BODY2GLOBAL/2
  Ground/1 -> mux3/1  "roll"
  Mux2/1 -> Mux1/2, Transformation_BODY2GLOBAL/1
  Discrete-Time Integrator/1 -> Mux5/1  "PosVEH wrt  GLOB"

== system TSR_Scenario_005_cs/Fiat_Bravo_1/Dynamics_Empty/STATE_Fiat_Bravo_1 ==
  State : Inport  SampleTime=TimeStep
  Bus Creator : BusCreator  Inputs=15  OutDataTypeStr=Bus: PRESCAN_STATEACTUATORDATA  NonVirtualBus=on
  Constant : Constant  Value=0
  Demux : Demux  Outputs=15
  Mux : Mux  Inputs=3
  Mux1 : Mux  Inputs=3
  Mux2 : Mux  Inputs=3
  iniBODYAngles wrtVEH [rad] : Constant  Value=Roll0  SampleTime=TimeStep
  iniBODYAngles wrtVEH [rad]1 : Constant  Value=Pitch0  SampleTime=TimeStep
  iniVEHAngles wrtGLOB [rad] : Constant  Value=Yaw0  SampleTime=TimeStep
  iniVEHposition wrtGLOB [m] : Constant  Value=x0  SampleTime=TimeStep
  iniVEHposition wrtGLOB [m]1 : Constant  Value=y0  SampleTime=TimeStep
  iniVEHposition wrtGLOB [m]2 : Constant  Value=z0  SampleTime=TimeStep
  state2FullState : PreScanSimulinkLibrary/state2FullState  SystemSampleTime=-1
  StateBus : Outport  OutDataTypeStr=Bus: PRESCAN_STATEACTUATORDATA
  wires:
  Mux2/1 -> state2FullState/4
  iniVEHAngles wrtGLOB [rad]/1 -> Mux2/3
  Mux1/1 -> state2FullState/3
  Constant/1 -> Mux2/1, Mux2/2, Mux1/3
  iniBODYAngles wrtVEH [rad]1/1 -> Mux1/2
  iniBODYAngles wrtVEH [rad]/1 -> Mux1/1
  Mux/1 -> state2FullState/2
  iniVEHposition wrtGLOB [m]2/1 -> Mux/3
  iniVEHposition wrtGLOB [m]/1 -> Mux/1
  iniVEHposition wrtGLOB [m]1/1 -> Mux/2
  Demux/15 -> Bus Creator/15  "AngularVelocityYaw"
  Demux/14 -> Bus Creator/14  "AngularVelocityPitch"
  Demux/13 -> Bus Creator/13  "AngularVelocityRoll"
  Demux/12 -> Bus Creator/12  "OrientationYaw"
  Demux/11 -> Bus Creator/11  "OrientationPitch"
  Demux/10 -> Bus Creator/10  "OrientationRoll"
  Demux/9 -> Bus Creator/9  "AccelerationZ"
  Demux/8 -> Bus Creator/8  "AccelerationY"
  Demux/7 -> Bus Creator/7  "AccelerationX"
  Demux/6 -> Bus Creator/6  "VelocityZ"
  Demux/5 -> Bus Creator/5  "VelocityY"
  Demux/4 -> Bus Creator/4  "VelocityX"
  Demux/3 -> Bus Creator/3  "PositionZ"
  Demux/2 -> Bus Creator/2  "PositionY"
  Demux/1 -> Bus Creator/1  "PositionX"
  state2FullState/1 -> Demux/1
  State/1 -> state2FullState/1
  Bus Creator/1 -> StateBus/1

== system TSR_Scenario_005_cs/Fiat_Bravo_1/SELF_Demux/compas converter ==
  rotz [rad] : Inport
  cart2compas : Subsystem
  rad2deg : Gain  Gain=180/pi
  heading [deg] : Outport
  wires:
  rad2deg/1 -> cart2compas/1(Angle [deg])
  rotz [rad]/1 -> rad2deg/1
  cart2compas/1(heading [deg]) -> heading [deg]/1

== system TSR_Scenario_005_cs/Fiat_Bravo_2/Dynamics_Empty/MuxState ==
  note: mode: Dynamics
  note: mode: Positioning
  note: mode: Dynamics
      | VelVEHICLE
      | wrt VEH
  note: AnglesVEHICLE
      | wrtGLOB
  note: For state mode 'Dynamic' positions
      | are not taken into account, as they
      | are computed by integrating velocity.
      | Click annotation for Help.
  x [m] : Inport  SampleTime=TimeStep
  y [m] : Inport  Port=2  SampleTime=TimeStep
  z [m] : Inport  Port=3  SampleTime=TimeStep
  dx [m/s] : Inport  Port=4  SampleTime=TimeStep
  dy [m/s] : Inport  Port=5  SampleTime=TimeStep
  dz [m/s] : Inport  Port=6  SampleTime=TimeStep
  R [rad] : Inport  Port=7  SampleTime=TimeStep
  P [rad] : Inport  Port=8  SampleTime=TimeStep
  Y [rad] : Inport  Port=9  SampleTime=TimeStep
  Constant : Constant  DisableCoverage=on  Value=positioningmode
  Discrete-Time Integrator : DiscreteIntegrator  SampleTime=TimeStep
  Ground : Ground
  Ground1 : Ground
  Mux1 : Mux  Inputs=[3 3]
  Mux2 : Mux  Inputs=3
  Mux3 : Mux  Inputs=3
  Mux4 : Mux  Inputs=3
  Mux5 : Mux  Inputs=[3 3]
  Mux6 : Mux  Inputs=[6 3]
  Switch : Switch  Threshold=0.5
  Transformation_BODY2GLOBAL : PreScanSimulinkLibrary/Simple_Vehicle_Dynamics/Chassis/MuxDynState/Transformation_BODY2GLOBAL
  mux3 : Mux  Inputs=3
  state : Outport
  wires:
  Constant/1 -> Switch/2
  Mux6/1 -> state/1
  Mux4/1 -> Mux1/1
  Mux5/1 -> Switch/3
  Mux1/1 -> Switch/1
  Switch/1 -> Mux6/1  "PosVeh wrt  GLOB"
  P [rad]/1 -> Mux3/2
  R [rad]/1 -> Mux3/1
  dz [m/s]/1 -> Mux2/3
  dy [m/s]/1 -> Mux2/2
  dx [m/s]/1 -> Mux2/1
  z [m]/1 -> Mux4/3
  y [m]/1 -> Mux4/2
  x [m]/1 -> Mux4/1
  Ground1/1 -> mux3/2  "pitch"
  Y [rad]/1 -> mux3/3, Mux3/3  "yaw"
  Mux3/1 -> Mux6/2
  Transformation_BODY2GLOBAL/1 -> Discrete-Time Integrator/1, Mux5/2  "VelVEH wrt  GLOB"
  mux3/1 -> Transformation_BODY2GLOBAL/2
  Ground/1 -> mux3/1  "roll"
  Mux2/1 -> Mux1/2, Transformation_BODY2GLOBAL/1
  Discrete-Time Integrator/1 -> Mux5/1  "PosVEH wrt  GLOB"

== system TSR_Scenario_005_cs/Fiat_Bravo_2/Dynamics_Empty/STATE_Fiat_Bravo_2 ==
  State : Inport  SampleTime=TimeStep
  Bus Creator : BusCreator  Inputs=15  OutDataTypeStr=Bus: PRESCAN_STATEACTUATORDATA  NonVirtualBus=on
  Constant : Constant  Value=0
  Demux : Demux  Outputs=15
  Mux : Mux  Inputs=3
  Mux1 : Mux  Inputs=3
  Mux2 : Mux  Inputs=3
  iniBODYAngles wrtVEH [rad] : Constant  Value=Roll0  SampleTime=TimeStep
  iniBODYAngles wrtVEH [rad]1 : Constant  Value=Pitch0  SampleTime=TimeStep
  iniVEHAngles wrtGLOB [rad] : Constant  Value=Yaw0  SampleTime=TimeStep
  iniVEHposition wrtGLOB [m] : Constant  Value=x0  SampleTime=TimeStep
  iniVEHposition wrtGLOB [m]1 : Constant  Value=y0  SampleTime=TimeStep
  iniVEHposition wrtGLOB [m]2 : Constant  Value=z0  SampleTime=TimeStep
  state2FullState : PreScanSimulinkLibrary/state2FullState  SystemSampleTime=-1
  StateBus : Outport  OutDataTypeStr=Bus: PRESCAN_STATEACTUATORDATA
  wires:
  Mux2/1 -> state2FullState/4
  iniVEHAngles wrtGLOB [rad]/1 -> Mux2/3
  Mux1/1 -> state2FullState/3
  Constant/1 -> Mux2/1, Mux2/2, Mux1/3
  iniBODYAngles wrtVEH [rad]1/1 -> Mux1/2
  iniBODYAngles wrtVEH [rad]/1 -> Mux1/1
  Mux/1 -> state2FullState/2
  iniVEHposition wrtGLOB [m]2/1 -> Mux/3
  iniVEHposition wrtGLOB [m]/1 -> Mux/1
  iniVEHposition wrtGLOB [m]1/1 -> Mux/2
  Demux/15 -> Bus Creator/15  "AngularVelocityYaw"
  Demux/14 -> Bus Creator/14  "AngularVelocityPitch"
  Demux/13 -> Bus Creator/13  "AngularVelocityRoll"
  Demux/12 -> Bus Creator/12  "OrientationYaw"
  Demux/11 -> Bus Creator/11  "OrientationPitch"
  Demux/10 -> Bus Creator/10  "OrientationRoll"
  Demux/9 -> Bus Creator/9  "AccelerationZ"
  Demux/8 -> Bus Creator/8  "AccelerationY"
  Demux/7 -> Bus Creator/7  "AccelerationX"
  Demux/6 -> Bus Creator/6  "VelocityZ"
  Demux/5 -> Bus Creator/5  "VelocityY"
  Demux/4 -> Bus Creator/4  "VelocityX"
  Demux/3 -> Bus Creator/3  "PositionZ"
  Demux/2 -> Bus Creator/2  "PositionY"
  Demux/1 -> Bus Creator/1  "PositionX"
  state2FullState/1 -> Demux/1
  State/1 -> state2FullState/1
  Bus Creator/1 -> StateBus/1

== system TSR_Scenario_005_cs/Fiat_Bravo_2/SELF_Demux/compas converter ==
  rotz [rad] : Inport
  cart2compas : Subsystem
  rad2deg : Gain  Gain=180/pi
  heading [deg] : Outport
  wires:
  rad2deg/1 -> cart2compas/1(Angle [deg])
  rotz [rad]/1 -> rad2deg/1
  cart2compas/1(heading [deg]) -> heading [deg]/1

== system TSR_Scenario_005_cs/Ford_Fiesta_1/SELF_Demux/compas converter ==
  rotz [rad] : Inport
  cart2compas : Subsystem
  rad2deg : Gain  Gain=180/pi
  heading [deg] : Outport
  wires:
  rad2deg/1 -> cart2compas/1(Angle [deg])
  rotz [rad]/1 -> rad2deg/1
  cart2compas/1(heading [deg]) -> heading [deg]/1

== system TSR_Scenario_005_cs/Ford_Fiesta_1/WheelDisplacement_Mux/WheelL0_Mux ==
  X [m] : Inport
  Y [m] : Inport  Port=2
  Z [m] : Inport  Port=3
  Roll [rad] : Inport  Port=4
  Pitch [rad] : Inport  Port=5
  Yaw [rad] : Inport  Port=6
  Bus Creator : BusCreator  Inputs=3  OutDataTypeStr=Bus: PRESCAN_XYZ_DATA
  Bus Creator1 : BusCreator  Inputs=3  OutDataTypeStr=Bus: PRESCAN_RPY_DATA
  Bus Creator2 : BusCreator  Inputs=2  OutDataTypeStr=Bus: PRESCAN_POSE_DATA
  Joint : Outport
  wires:
  Yaw [rad]/1 -> Bus Creator1/3  "Yaw"
  Bus Creator1/1 -> Bus Creator2/2  "ORIENTATION"
  Bus Creator/1 -> Bus Creator2/1  "POSITION"
  X [m]/1 -> Bus Creator/1  "X"
  Y [m]/1 -> Bus Creator/2  "Y"
  Z [m]/1 -> Bus Creator/3  "Z"
  Bus Creator2/1 -> Joint/1
  Roll [rad]/1 -> Bus Creator1/1  "Roll"
  Pitch [rad]/1 -> Bus Creator1/2  "Pitch"

== system TSR_Scenario_005_cs/Ford_Fiesta_1/WheelDisplacement_Mux/WheelL1_Mux ==
  X [m] : Inport
  Y [m] : Inport  Port=2
  Z [m] : Inport  Port=3
  Roll [rad] : Inport  Port=4
  Pitch [rad] : Inport  Port=5
  Yaw [rad] : Inport  Port=6
  Bus Creator : BusCreator  Inputs=3  OutDataTypeStr=Bus: PRESCAN_XYZ_DATA
  Bus Creator1 : BusCreator  Inputs=3  OutDataTypeStr=Bus: PRESCAN_RPY_DATA
  Bus Creator2 : BusCreator  Inputs=2  OutDataTypeStr=Bus: PRESCAN_POSE_DATA
  Joint : Outport
  wires:
  Yaw [rad]/1 -> Bus Creator1/3  "Yaw"
  Bus Creator1/1 -> Bus Creator2/2  "ORIENTATION"
  Bus Creator/1 -> Bus Creator2/1  "POSITION"
  X [m]/1 -> Bus Creator/1  "X"
  Y [m]/1 -> Bus Creator/2  "Y"
  Z [m]/1 -> Bus Creator/3  "Z"
  Bus Creator2/1 -> Joint/1
  Roll [rad]/1 -> Bus Creator1/1  "Roll"
  Pitch [rad]/1 -> Bus Creator1/2  "Pitch"

== system TSR_Scenario_005_cs/Ford_Fiesta_1/WheelDisplacement_Mux/WheelR0_Mux ==
  X [m] : Inport
  Y [m] : Inport  Port=2
  Z [m] : Inport  Port=3
  Roll [rad] : Inport  Port=4
  Pitch [rad] : Inport  Port=5
  Yaw [rad] : Inport  Port=6
  Bus Creator : BusCreator  Inputs=3  OutDataTypeStr=Bus: PRESCAN_XYZ_DATA
  Bus Creator1 : BusCreator  Inputs=3  OutDataTypeStr=Bus: PRESCAN_RPY_DATA
  Bus Creator2 : BusCreator  Inputs=2  OutDataTypeStr=Bus: PRESCAN_POSE_DATA
  Joint : Outport
  wires:
  Yaw [rad]/1 -> Bus Creator1/3  "Yaw"
  Bus Creator1/1 -> Bus Creator2/2  "ORIENTATION"
  Bus Creator/1 -> Bus Creator2/1  "POSITION"
  X [m]/1 -> Bus Creator/1  "X"
  Y [m]/1 -> Bus Creator/2  "Y"
  Z [m]/1 -> Bus Creator/3  "Z"
  Bus Creator2/1 -> Joint/1
  Roll [rad]/1 -> Bus Creator1/1  "Roll"
  Pitch [rad]/1 -> Bus Creator1/2  "Pitch"

== system TSR_Scenario_005_cs/Ford_Fiesta_1/WheelDisplacement_Mux/WheelR1_Mux ==
  X [m] : Inport
  Y [m] : Inport  Port=2
  Z [m] : Inport  Port=3
  Roll [rad] : Inport  Port=4
  Pitch [rad] : Inport  Port=5
  Yaw [rad] : Inport  Port=6
  Bus Creator : BusCreator  Inputs=3  OutDataTypeStr=Bus: PRESCAN_XYZ_DATA
  Bus Creator1 : BusCreator  Inputs=3  OutDataTypeStr=Bus: PRESCAN_RPY_DATA
  Bus Creator2 : BusCreator  Inputs=2  OutDataTypeStr=Bus: PRESCAN_POSE_DATA
  Joint : Outport
  wires:
  Yaw [rad]/1 -> Bus Creator1/3  "Yaw"
  Bus Creator1/1 -> Bus Creator2/2  "ORIENTATION"
  Bus Creator/1 -> Bus Creator2/1  "POSITION"
  X [m]/1 -> Bus Creator/1  "X"
  Y [m]/1 -> Bus Creator/2  "Y"
  Z [m]/1 -> Bus Creator/3  "Z"
  Bus Creator2/1 -> Joint/1
  Roll [rad]/1 -> Bus Creator1/1  "Roll"
  Pitch [rad]/1 -> Bus Creator1/2  "Pitch"

== system TSR_Scenario_005_cs/FullCurtainSidedTrailer_1/Dynamics_Empty/MuxState ==
  note: mode: Dynamics
  note: mode: Positioning
  note: mode: Dynamics
      | VelVEHICLE
      | wrt VEH
  note: AnglesVEHICLE
      | wrtGLOB
  note: For state mode 'Dynamic' positions
      | are not taken into account, as they
      | are computed by integrating velocity.
      | Click annotation for Help.
  x [m] : Inport  SampleTime=TimeStep
  y [m] : Inport  Port=2  SampleTime=TimeStep
  z [m] : Inport  Port=3  SampleTime=TimeStep
  dx [m/s] : Inport  Port=4  SampleTime=TimeStep
  dy [m/s] : Inport  Port=5  SampleTime=TimeStep
  dz [m/s] : Inport  Port=6  SampleTime=TimeStep
  R [rad] : Inport  Port=7  SampleTime=TimeStep
  P [rad] : Inport  Port=8  SampleTime=TimeStep
  Y [rad] : Inport  Port=9  SampleTime=TimeStep
  Constant : Constant  DisableCoverage=on  Value=positioningmode
  Discrete-Time Integrator : DiscreteIntegrator  SampleTime=TimeStep
  Ground : Ground
  Ground1 : Ground
  Mux1 : Mux  Inputs=[3 3]
  Mux2 : Mux  Inputs=3
  Mux3 : Mux  Inputs=3
  Mux4 : Mux  Inputs=3
  Mux5 : Mux  Inputs=[3 3]
  Mux6 : Mux  Inputs=[6 3]
  Switch : Switch  Threshold=0.5
  Transformation_BODY2GLOBAL : PreScanSimulinkLibrary/Simple_Vehicle_Dynamics/Chassis/MuxDynState/Transformation_BODY2GLOBAL
  mux3 : Mux  Inputs=3
  state : Outport
  wires:
  Constant/1 -> Switch/2
  Mux6/1 -> state/1
  Mux4/1 -> Mux1/1
  Mux5/1 -> Switch/3
  Mux1/1 -> Switch/1
  Switch/1 -> Mux6/1  "PosVeh wrt  GLOB"
  P [rad]/1 -> Mux3/2
  R [rad]/1 -> Mux3/1
  dz [m/s]/1 -> Mux2/3
  dy [m/s]/1 -> Mux2/2
  dx [m/s]/1 -> Mux2/1
  z [m]/1 -> Mux4/3
  y [m]/1 -> Mux4/2
  x [m]/1 -> Mux4/1
  Ground1/1 -> mux3/2  "pitch"
  Y [rad]/1 -> mux3/3, Mux3/3  "yaw"
  Mux3/1 -> Mux6/2
  Transformation_BODY2GLOBAL/1 -> Discrete-Time Integrator/1, Mux5/2  "VelVEH wrt  GLOB"
  mux3/1 -> Transformation_BODY2GLOBAL/2
  Ground/1 -> mux3/1  "roll"
  Mux2/1 -> Mux1/2, Transformation_BODY2GLOBAL/1
  Discrete-Time Integrator/1 -> Mux5/1  "PosVEH wrt  GLOB"
